simulink model "DSP_Block_Lab3"  (R2016a)
settings: Solver=VariableStepAuto  StartTime=0.0  StopTime=50.0  RelTol=1e-3
libraries: dspsrcs4 x2
settings Model: Creator=Sheldon1203G  LastModifiedBy=Sheldon1203G

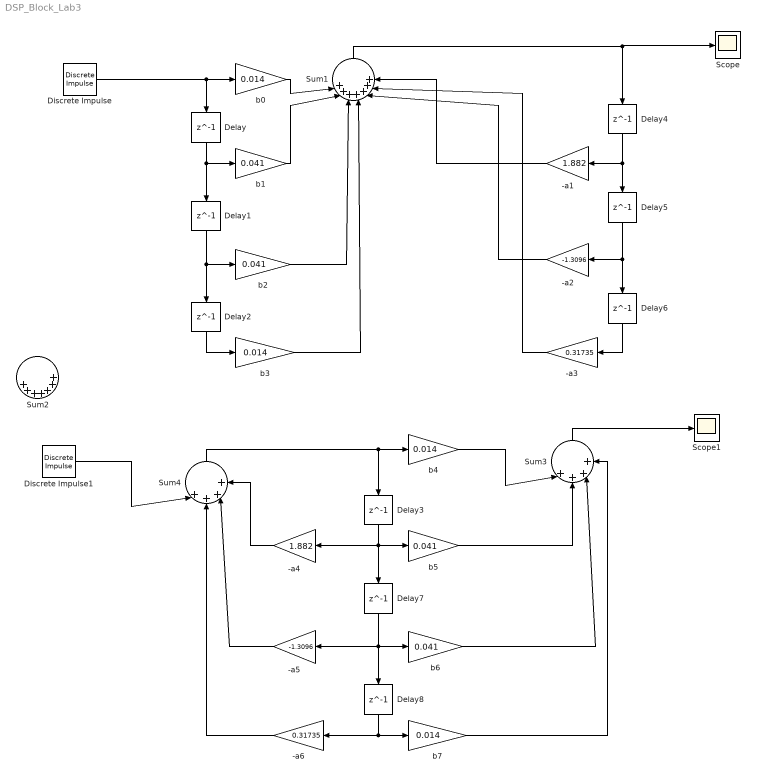
== system DSP_Block_Lab3 ==
  -a1 : Gain  Gain=1.882
  -a2 : Gain  Gain=-1.3096
  -a3 : Gain  Gain=0.31735
  -a4 : Gain  Gain=1.882
  -a5 : Gain  Gain=-1.3096
  -a6 : Gain  Gain=0.31735
  Delay{,1..8} (9 alike) : Delay  DelayLength=1  InitialCondition=0
  Discrete Impulse : dspsrcs4/Discrete  Impulse  Delay=0  SampleTime=1  FrameSample=1  OutputFrames=off  dataType=double  isSigned=on  wordLen=16  udDataType=sfix(16)  fracBitsMode=Best precision  numFracBits=15  OutDataTypeStr=double  LastOutDataTypeStr=double
  Discrete Impulse1 : dspsrcs4/Discrete  Impulse  Delay=0  SampleTime=1  FrameSample=1  OutputFrames=off  dataType=double  isSigned=on  wordLen=16  udDataType=sfix(16)  fracBitsMode=Best precision  numFracBits=15  OutDataTypeStr=double  LastOutDataTypeStr=double
  Scope : Scope
  Scope1 : Scope
  Sum1 : Sum  Inputs=|+++++++
  Sum2 : Sum  Inputs=|+++++++
  Sum3 : Sum  Inputs=|++++
  Sum4 : Sum  Inputs=|++++
  b{0,3..4,7} (4 alike) : Gain  Gain=0.014
  b{1..2,5..6} (4 alike) : Gain  Gain=0.041
  wires:
  Delay/1 -> Delay1/1, b1/1
  Discrete Impulse/1 -> Delay/1, b0/1
  Delay2/1 -> b3/1
  Delay1/1 -> Delay2/1, b2/1
  b0/1 -> Sum1/1
  b1/1 -> Sum1/2
  b2/1 -> Sum1/3
  b3/1 -> Sum1/4
  Sum1/1 -> Delay4/1, Scope/1
  Delay4/1 -> Delay5/1, -a1/1
  Delay5/1 -> Delay6/1, -a2/1
  Delay6/1 -> -a3/1
  -a2/1 -> Sum1/5
  -a1/1 -> Sum1/7
  -a3/1 -> Sum1/6
  Delay3/1 -> -a4/1, Delay7/1, b5/1
  Delay8/1 -> -a6/1, b7/1
  Delay7/1 -> -a5/1, Delay8/1, b6/1
  b4/1 -> Sum3/1
  b5/1 -> Sum3/2
  b6/1 -> Sum3/3
  b7/1 -> Sum3/4
  Sum3/1 -> Scope1/1
  Sum4/1 -> Delay3/1, b4/1
  Discrete Impulse1/1 -> Sum4/1
  -a4/1 -> Sum4/4
  -a5/1 -> Sum4/3
  -a6/1 -> Sum4/2
